simulink model "model_response"  (R2024a)
settings: Solver=VariableStepAuto  StartTime=0.0  StopTime=10.0  RelTol=1e-3
values from neighbouring files (symbols this model uses):
  C = K * s    [comp_select.m]    (also in compensation.m; compensation_rework.m; compensator_optimization.m = K * C1 * C2 * C3 * notch_filter_ar * notch_filter_r; loopgain.m = C*C_set(i))
  G = DC_gain * G_resonance * 1 / (s + pole_1) * 1 / (s + pole_2)    [carson.m]    (also in compensation.m; compensation_rework.m; compensator_optimization.m; owen.m)
undefined symbols (not defined in the file or in its folder): sinStepBool
settings Model: Creator=carso  LastModifiedBy=dunni

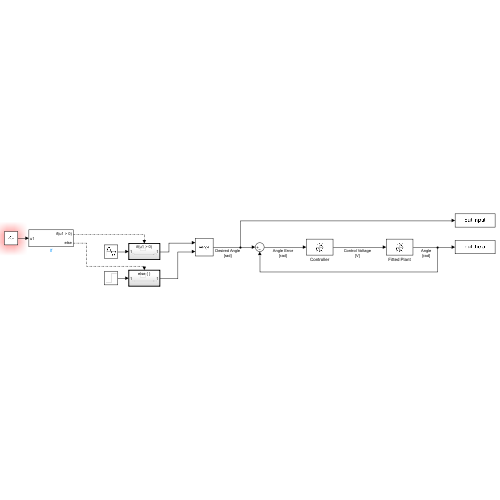
[thumbnail: Simulink's stored preview of the top-level diagram]
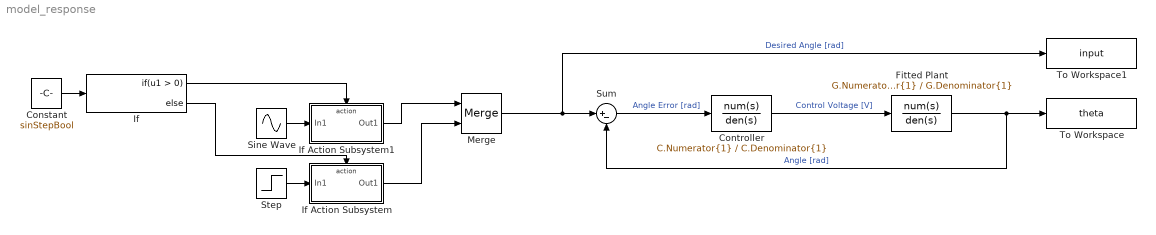
== system model_response ==
  Constant : Constant  Value=sinStepBool
  Controller : TransferFcn  Numerator=C.Numerator{1}  Denominator=C.Denominator{1}
  Fitted Plant : TransferFcn  Numerator=G.Numerator{1}  Denominator=G.Denominator{1}
  If : If
  If Action Subsystem : Subsystem  TreatAsAtomicUnit=on
  If Action Subsystem1 : Subsystem  TreatAsAtomicUnit=on
  Merge : Merge
  Sine Wave : Sin  SampleTime=0
  Step : Step  SampleTime=0
  Sum : Sum  Inputs=|+-
  To Workspace : ToWorkspace  VariableName=theta  SaveFormat=Timeseries  SampleTime=-1
  To Workspace1 : ToWorkspace  VariableName=input  SaveFormat=Timeseries  SampleTime=-1
  wires:
  Controller/1 -> Fitted Plant/1  "Control Voltage [V]"
  Sum/1 -> Controller/1  "Angle Error [rad]"
  Fitted Plant/1 -> Sum/2, To Workspace/1  "Angle [rad]"
  Merge/1 -> To Workspace1/1, Sum/1  "Desired Angle [rad]"
  If/2 -> If Action Subsystem/Action
  If/1 -> If Action Subsystem1/Action
  If Action Subsystem1/1(Out1) -> Merge/1
  If Action Subsystem/1(Out1) -> Merge/2
  Constant/1 -> If/1
  Step/1 -> If Action Subsystem/1(In1)
  Sine Wave/1 -> If Action Subsystem1/1(In1)

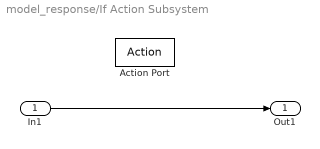
== system model_response/If Action Subsystem ==
  In1 : Inport
  Action Port : ActionPort  ActionPortLabel=else
  Out1 : Outport
  wires:
  In1/1 -> Out1/1

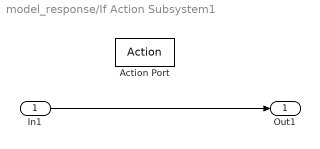
== system model_response/If Action Subsystem1 ==
  In1 : Inport
  Action Port : ActionPort  ActionPortLabel=if(u1 > 0)
  Out1 : Outport
  wires:
  In1/1 -> Out1/1
